simulink model "COSTEP_Exergy"  (R2024b)
settings: Solver=FixedStepAuto  StartTime=0.0  StopTime=25  FixedStep=1/3600  RelTol=1e-3
model workspace (MAT data in the model file):
  AD : Simulink.Parameter (value not decoded)
  AG : Simulink.Parameter (value not decoded)
  AH : Simulink.Parameter (value not decoded)
  AV : Simulink.Parameter (value not decoded)
  AVP : Simulink.Parameter (value not decoded)
  BCHL : Simulink.Parameter (value not decoded)
  BCHV : Simulink.Parameter (value not decoded)
  BD : Simulink.Parameter (value not decoded)
  BDIST : Simulink.Parameter (value not decoded)
  BG : Simulink.Parameter (value not decoded)
  BH : Simulink.Parameter (value not decoded)
  BVP : Simulink.Parameter (value not decoded)
  CD : Simulink.Parameter (value not decoded)
  CDIST : Simulink.Parameter (value not decoded)
  CG : Simulink.Parameter (value not decoded)
  CH : Simulink.Parameter (value not decoded)
  CVP : Simulink.Parameter (value not decoded)
  DDIST : Simulink.Parameter (value not decoded)
  DIST_CONST : Simulink.Parameter (value not decoded)
  ISV : Simulink.Parameter (value not decoded)
  TLAST : Simulink.Parameter (value not decoded)
  TNEXT : Simulink.Parameter (value not decoded)
  XMW : Simulink.Parameter (value not decoded)
  XNS : Simulink.Parameter (value not decoded)
  XNS2 : Simulink.Parameter (value not decoded)
  XNS3 : Simulink.Parameter (value not decoded)
  XNSADD : Simulink.Parameter (value not decoded)
  XNSE : Simulink.Parameter (value not decoded)
symbols that are objects in the model workspace (value not decoded): AD, AG, AH, AV, AVP, BD, BG, BH, BVP, CD, CG, CH, CVP, XMW, XNS, XNS2, XNS3, XNSE
undefined symbols (not defined in the file or in its folder): magnitude, msgbox, SETPT, XMEAS, XMV
libraries: mylib x403, dspindex x31
(part 2 of 13)

== system COSTEP_Exergy/Condenser/Position of Valve 11 % ==
  Bus Selector : BusSelector  OutputSignals=XMV(11)
  Bus Selector1 : BusSelector  OutputSignals=IDV(15)
  Constant : Constant  Value=49
  Control valve : mylib/Control valve  SystemSampleTime=-1  VariantActivationTime=update diagram  AllowFlexibleInterface=on  Latency=0  AutoFrameSizeCalculation=off
  Divide : Product  Inputs=*/
  Initial state variable : mylib/Initial state variable
  Integration : mylib/Integration  SystemSampleTime=-1  VariantActivationTime=update diagram  AllowFlexibleInterface=on  Latency=0  AutoFrameSizeCalculation=off
  Subtract : Sum  Inputs=+-
  VTAU(11) : Constant  Value=5/3600
  "YY(49) " : Outport  PortDimensions=1  VectorParamsAs1DForOutWhenUnconnected=off
  wires:
  Integration/1 -> "YY(49) "/1, Subtract/2  "VPOS(11)"
  Subtract/1 -> Divide/1
  Control valve/1 -> Subtract/1
  VTAU(11)/1 -> Divide/2
  Divide/1 -> Integration/1
  Initial state variable/1 -> Integration/2
  [XMV] -> Bus Selector/1
  Bus Selector/1 -> Control valve/1  "<XMV(11)>"
  Bus Selector1/1 -> Control valve/2  "<IDV(15)>"
  [IDV] -> Bus Selector1/1
  Constant/1 -> Initial state variable/1

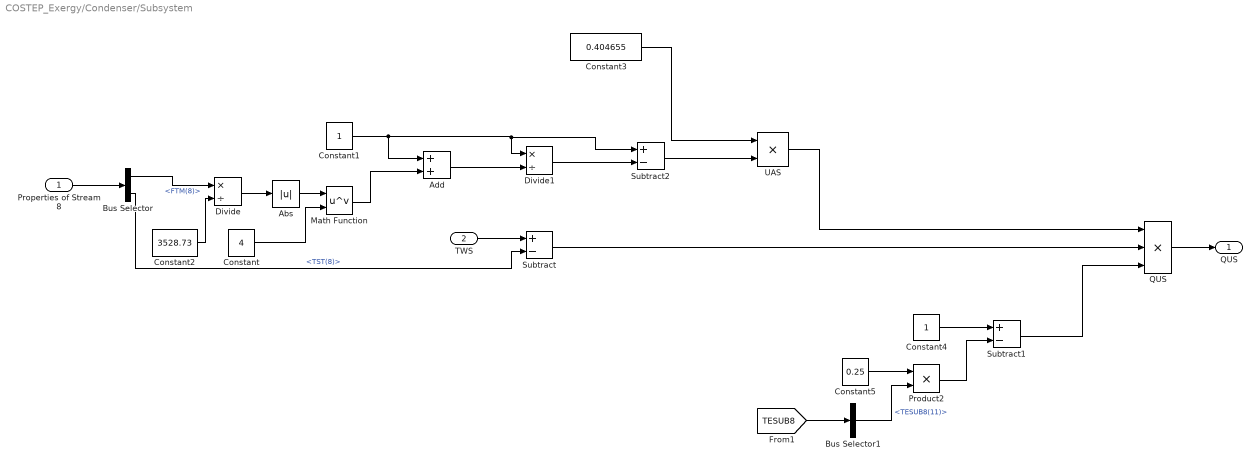
== system COSTEP_Exergy/Condenser/Subsystem ==
  Properties of Stream 8 : Inport
  TWS : Inport  Port=2
  Abs : Abs  SaturateOnIntegerOverflow=off
  Add : Sum
  Bus Selector : BusSelector  OutputSignals=FTM(8),TST(8)
  Bus Selector1 : BusSelector  OutputSignals=signal2.TESUB8(11)
  Constant : Constant  Value=4
  Constant1 : Constant
  Constant2 : Constant  Value=3528.73
  Constant3 : Constant  Value=0.404655
  Constant4 : Constant
  Constant5 : Constant  Value=0.25
  Divide : Product  Inputs=*/
  Divide1 : Product  Inputs=*/
  Math Function : Math  Operator=pow  SignedPower=on
  Product2 : Product
  QUS : Product  Inputs=3
  Subtract : Sum  Inputs=+-
  Subtract1 : Sum  Inputs=+-
  Subtract2 : Sum  Inputs=+-
  UAS : Product
  "QUS " : Outport  VectorParamsAs1DForOutWhenUnconnected=off
  wires:
  Product2/1 -> Subtract1/2
  Constant4/1 -> Subtract1/1
  UAS/1 -> QUS/1
  Properties of Stream 8/1 -> Bus Selector/1
  Add/1 -> Divide1/2
  Constant2/1 -> Divide/2
  Math Function/1 -> Add/2
  Constant1/1 -> Subtract2/1, Divide1/1, Add/1
  Subtract1/1 -> QUS/3
  Constant/1 -> Math Function/2
  Bus Selector/2 -> Subtract/2  "<TST(8)>"
  Bus Selector/1 -> Divide/1  "<FTM(8)>"
  Divide1/1 -> Subtract2/2
  Divide/1 -> Abs/1
  Subtract/1 -> QUS/2
  Constant3/1 -> UAS/1
  Bus Selector1/1 -> Product2/2  "<TESUB8(11)>"
  Subtract2/1 -> UAS/2
  Constant5/1 -> Product2/1
  Abs/1 -> Math Function/1
  [TESUB8] -> Bus Selector1/1
  TWS/1 -> Subtract/1
  QUS/1 -> "QUS "/1

== system COSTEP_Exergy/Condenser/VRNG(11) Max flow of water through valve Gallons per minute ==
  Bus Selector : BusSelector  OutputSignals=signal3.TESUB8(20)
  VRNG(11) : Outport  PortDimensions=1  VectorParamsAs1DForOutWhenUnconnected=off
  wires:
  [TESUB8] -> Bus Selector/1
  Bus Selector/1 -> VRNG(11)/1  "<TESUB8(20)>"

== system COSTEP_Exergy/Control Mode/Braatz ==
  XMEAS : Inport
  " " : Subsystem  mask{Parameter1=XMV(1), Parameter2=XMEAS(2), SETPT1=3664.0, GAIN1=1, SI1=3/3600, HIGH1=5811, Parameter1_copy=SETPT(1), Parameter2_copy=XMEAS(26), SETPT14=6.8820, GAIN14=8.3, TAUI14=3168.0/3600, SI14=360/3600, HIGH14=100}
      mask prompts: Parameter1 "Manipulated Variable"; Parameter2 "Process Variable"; SETPT1 "Setpoint"; GAIN1 "Controller Gain"; SI1 "Sampling Interval"; HIGH1 "High Limit"; Parameter1_copy "Manipulated Variable"; Parameter2_copy "Process Variable"; SETPT14 "Setpoint"; GAIN14 "Controller Gain"; TAUI14 "Integral Time Constant"; SI14 "Sampling Interval"; HIGH14 "High Limit"
      mask DialogControl DescGroupVar Prompt: Control Variables
      mask DialogControl DescTextVar Prompt: Enter the control variables needed
      mask DialogControl ParameterGroupVar Prompt: Control 1
      mask DialogControl Container3 Prompt: Control 14
  " 1" : Subsystem  mask{Parameter1=XMV(2), Parameter2=XMEAS(3), SETPT2=4509.3, GAIN2=1.0, SI2=3/3600, HIGH2=8354, Parameter1_copy=SETPT(2), Parameter2_copy=XMEAS(27), SETPT15=18.776, GAIN15=2.37, TAUI15=5069/3600, SI15=360/3600, HIGH15=100}
      mask prompts: Parameter1 "Manipulated Variable"; Parameter2 "Process Variable"; SETPT2 "Setpoint"; GAIN2 "Controller Gain"; SI2 "Sampling Interval"; HIGH2 "High Limit"; Parameter1_copy "Manipulated Variable"; Parameter2_copy "Process Variable"; SETPT15 "Setpoint"; GAIN15 "Controller Gain"; TAUI15 "Integral Time Constant"; SI15 "Sampling Interval"; HIGH15 "High Limit"
      mask DialogControl DescGroupVar Prompt: Control Variables
      mask DialogControl DescTextVar Prompt: Enter the control variables needed
      mask DialogControl ParameterGroupVar Prompt: Control 2
      mask DialogControl Container3 Prompt: Control 15
  " 10" : Subsystem  mask{Parameter1=XMV(6), Parameter2=XMEAS(10), SETPT6=0.33712, GAIN6=1.22, SI6=3/3600, HIGH6=1, Parameter1_copy=SETPT(6), Parameter2_copy=XMEAS(30), SETPT19=13.823, GAIN19=-83.2/5/3, TAUI19=6336/3600, SI19=360/3600, HIGH19=26}
      mask prompts: Parameter1 "Manipulated Variable"; Parameter2 "Process Variable"; SETPT6 "Setpoint"; GAIN6 "Controller Gain"; SI6 "Sampling Interval"; HIGH6 "High Limit"; Parameter1_copy "Manipulated Variable"; Parameter2_copy "Process Variable"; SETPT19 "Setpoint"; GAIN19 "Controller Gain"; TAUI19 "Integral Time Constant"; SI19 "Sampling Interval"; HIGH19 "High Limit"
      mask DialogControl DescGroupVar Prompt: Control Variables
      mask DialogControl DescTextVar Prompt: Enter the control variables needed
      mask DialogControl ParameterGroupVar Prompt: Control 6
      mask DialogControl Container3 Prompt: Control 19
  " 2" : Subsystem  mask{Parameter1=XMV(3), Parameter2=XMEAS(1), SETPT3=0.25052, GAIN3=1.0, SI3=3/3600, HIGH3=1.017, Parameter1_copy=SETPT(3), Parameter2_copy=XMEAS(23), SETPT13=32.188, GAIN13=18, TAUI13=3168.0/3600, SI13=360/3600, HIGH13=100}
      mask prompts: Parameter1 "Manipulated Variable"; Parameter2 "Process Variable"; SETPT3 "Setpoint"; GAIN3 "Controller Gain"; SI3 "Sampling Interval"; HIGH3 "High Limit"; Parameter1_copy "Manipulated Variable"; Parameter2_copy "Process Variable"; SETPT13 "Setpoint"; GAIN13 "Controller Gain"; TAUI13 "Integral Time Constant"; SI13 "Sampling Interval"; HIGH13 "High Limit"
      mask DialogControl DescGroupVar Prompt: Control Variables
      mask DialogControl DescTextVar Prompt: Enter the control variables needed
      mask DialogControl ParameterGroupVar Prompt: Control 3
      mask DialogControl Container3 Prompt: Control 13
  " 3" : Subsystem  mask{Parameter1=XMV(4), Parameter2=XMEAS(4), SETPT4=9.3477, GAIN4=1.0, SI4=3/3600, HIGH4=15.25, Parameter1_copy=SETPT(4), Parameter2_copy=XMEAS(8), SETPT17=75, GAIN17=11.1/10, TAUI17=3168.0/3600, SI17=3/3600, HIGH17=50}
      mask prompts: Parameter1 "Manipulated Variable"; Parameter2 "Process Variable"; SETPT4 "Setpoint"; GAIN4 "Controller Gain"; SI4 "Sampling Interval"; HIGH4 "High Limit"; Parameter1_copy "Manipulated Variable"; Parameter2_copy "Process Variable"; SETPT17 "Setpoint"; GAIN17 "Controller Gain"; TAUI17 "Integral Time Constant"; SI17 "Sampling Interval"; HIGH17 "High Limit"
      mask DialogControl DescGroupVar Prompt: Control Variables
      mask DialogControl DescTextVar Prompt: Enter the control variables needed
      mask DialogControl ParameterGroupVar Prompt: Control 4
      mask DialogControl Container3 Prompt: Control 17
  " 4" : Subsystem  mask{Parameter1_copy=XMV(5), Parameter2_copy=XMEAS(5), SETPT5=26.902, GAIN5=-0.083, TAUI5=1/3600, SI5=3/3600, HIGH5=53}
      mask prompts: Parameter1_copy "Manipulated Variable"; Parameter2_copy "Process Variable"; SETPT5 "Setpoint"; GAIN5 "Controller Gain"; TAUI5 "Integral Time Constant"; SI5 "Sampling Interval"; HIGH5 "High Limit"
      mask DialogControl DescGroupVar Prompt: Control Variables
      mask DialogControl DescTextVar Prompt: Enter the control variables needed
      mask DialogControl Container3 Prompt: Control 5
  " 5" : Subsystem  mask{Parameter1_copy=XMV(7), Parameter2_copy=XMEAS(12), SETPT7=50, GAIN7=-2.06, SI7=3/3600, HIGH7=70}
      mask prompts: Parameter1_copy "Manipulated Variable"; Parameter2_copy "Process Variable"; SETPT7 "Setpoint"; GAIN7 "Controller Gain"; SI7 "Sampling Interval"; HIGH7 "High Limit"
      mask DialogControl DescGroupVar Prompt: Control Variables
      mask DialogControl DescTextVar Prompt: Enter the control variables needed
      mask DialogControl Container3 Prompt: Control 7
  " 6" : Subsystem  mask{Parameter1_copy=XMV(8), Parameter2_copy=XMEAS(15), SETPT8=50, GAIN8=-1.62, SI8=3/3600, HIGH8=70}
      mask prompts: Parameter1_copy "Manipulated Variable"; Parameter2_copy "Process Variable"; SETPT8 "Setpoint"; GAIN8 "Controller Gain"; SI8 "Sampling Interval"; HIGH8 "High Limit"
      mask DialogControl DescGroupVar Prompt: Control Variables
      mask DialogControl DescTextVar Prompt: Enter the control variables needed
      mask DialogControl Container3 Prompt: Control 8
  " 7" : Subsystem  mask{Parameter1_copy=XMV(11), Parameter2_copy=XMEAS(17), SETPT11=22.949, GAIN11=1.09, TAUI11=2600/3600, SI11=3/3600, HIGH11=46}
      mask prompts: Parameter1_copy "Manipulated Variable"; Parameter2_copy "Process Variable"; SETPT11 "Setpoint"; GAIN11 "Controller Gain"; TAUI11 "Integral Time Constant"; SI11 "Sampling Interval"; HIGH11 "High Limit"
      mask DialogControl DescGroupVar Prompt: Control Variables
      mask DialogControl DescTextVar Prompt: Enter the control variables needed
      mask DialogControl Container3 Prompt: Control 11
  " 8" : Subsystem  mask{Parameter1=XMV(10), Parameter2=XMEAS(21), SETPT10=94.599, GAIN10=-0.156*10, TAUI10=1452/3600, SI10=3/3600, HIGH10=150, Parameter1_copy=SETPT(10), Parameter2_copy=XMEAS(9), SETPT18=120.4, GAIN18=2.83*10, TAUI18=982/3600, SI18=3/3600, HIGH18=150}
      mask prompts: Parameter1 "Manipulated Variable"; Parameter2 "Process Variable"; SETPT10 "Setpoint"; GAIN10 "Controller Gain"; TAUI10 "Integral Time Constant"; SI10 "Sampling Interval"; HIGH10 "High Limit"; Parameter1_copy "Manipulated Variable"; Parameter2_copy "Process Variable"; SETPT18 "Setpoint"; GAIN18 "Controller Gain"; TAUI18 "Integral Time Constant"; SI18 "Sampling Interval"; HIGH18 "High Limit"
      mask DialogControl DescGroupVar Prompt: Control Variables
      mask DialogControl DescTextVar Prompt: Enter the control variables needed
      mask DialogControl ParameterGroupVar Prompt: Control 10
      mask DialogControl Container3 Prompt: Control 18
  " 9" : Subsystem  mask{Parameter1=XMV(9), Parameter2=XMEAS(19), SETPT9=230.31, GAIN9=0.41, SI9=3/3600, HIGH9=460, Parameter1_copy=SETPT(9), Parameter2_copy=XMEAS(18), SETPT16=65.731, GAIN16=1.69/10, TAUI16=236/3600, SI16=3/3600, HIGH16=130, Parameter1_copy_copy=SETPT(16), Parameter2_copy_copy=XMEAS(38), SETPT20=0.83570, GAIN20=-16.3/5, TAUI20=12408/3600, SI20=900/3600, HIGH20=1.6}
      mask prompts: Parameter1 "Manipulated Variable"; Parameter2 "Process Variable"; SETPT9 "Setpoint"; GAIN9 "Controller Gain"; SI9 "Sampling Interval"; HIGH9 "High Limit"; Parameter1_copy "Manipulated Variable"; Parameter2_copy "Process Variable"; SETPT16 "Setpoint"; GAIN16 "Controller Gain"; TAUI16 "Integral Time Constant"; SI16 "Sampling Interval"; HIGH16 "High Limit"; Parameter1_copy_copy "Manipulated Variable"; Parameter2_copy_copy "Process Variable"; SETPT20 "Setpoint"; GAIN20 "Controller Gain"; TAUI20 "Integral Time Constant"; SI20 "Sampling Interval"; HIGH20 "High Limit"
      mask DialogControl DescGroupVar Prompt: Control Variables
      mask DialogControl DescTextVar Prompt: Enter the control variables needed
      mask DialogControl ParameterGroupVar Prompt: Control 9
      mask DialogControl Container3 Prompt: Control 16
      mask DialogControl Container3_copy Prompt: Control 20
  Bus Creator : BusCreator  Inputs=12
  Constant11 : Constant  Value=XMV12_0
  XMV : Outport  VectorParamsAs1DForOutWhenUnconnected=off
  wires:
  " "/1(XMV(1)) -> Bus Creator/1  "XMV(1)"
  " 1"/1(XMV(2)) -> Bus Creator/2  "XMV(2)"
  " 2"/1(XMV(3)) -> Bus Creator/3  "XMV(3)"
  " 3"/1(XMV(4)) -> Bus Creator/4  "XMV(4)"
  " 4"/1(XMV(5)) -> Bus Creator/5  "XMV(5)"
  " 10"/1(XMV(6)) -> Bus Creator/6  "XMV(6)"
  " 5"/1(XMV(7)) -> Bus Creator/7  "XMV(7)"
  " 6"/1(XMV(8)) -> Bus Creator/8  "XMV(8)"
  " 9"/1(XMV(9)) -> Bus Creator/9  "XMV(9)"
  " 8"/1(XMV(10)) -> Bus Creator/10  "XMV(10)"
  " 7"/1(XMV(11)) -> Bus Creator/11  "XMV(11)"
  Constant11/1 -> Bus Creator/12  "XMV(12)"
  Bus Creator/1 -> XMV/1
  XMEAS/1 -> " 5"/1(XMEAS), " 9"/1(XMEAS), " 8"/1(XMEAS), " 7"/1(XMEAS), " 6"/1(XMEAS), " 10"/1(XMEAS), " 4"/1(XMEAS), " 3"/1(XMEAS), " 2"/1(XMEAS), " 1"/1(XMEAS), " "/1(XMEAS)

== system COSTEP_Exergy/Control Mode/Custom Controller ==
  Bus Creator : BusCreator  Inputs=12
  Constant : Constant  Value=XMV1_0
  Constant1 : Constant  Value=XMV2_0
  Constant10 : Constant  Value=XMV11_0
  Constant11 : Constant  Value=XMV12_0
  Constant2 : Constant  Value=XMV3_0
  Constant3 : Constant  Value=XMV4_0
  Constant4 : Constant  Value=XMV5_0
  Constant5 : Constant  Value=XMV6_0
  Constant6 : Constant  Value=XMV7_0
  Constant7 : Constant  Value=XMV8_0
  Constant8 : Constant  Value=XMV9_0
  Constant9 : Constant  Value=XMV10_0
  XMV : Outport  VectorParamsAs1DForOutWhenUnconnected=off
  wires:
  Constant5/1 -> Bus Creator/6  "XMV(6)"
  Constant1/1 -> Bus Creator/2  "XMV(2)"
  Constant4/1 -> Bus Creator/5  "XMV(5)"
  Constant3/1 -> Bus Creator/4  "XMV(4)"
  Constant2/1 -> Bus Creator/3  "XMV(3)"
  Constant11/1 -> Bus Creator/12  "XMV(12)"
  Constant10/1 -> Bus Creator/11  "XMV(11)"
  Constant/1 -> Bus Creator/1  "XMV(1)"
  Constant9/1 -> Bus Creator/10  "XMV(10)"
  Constant8/1 -> Bus Creator/9  "XMV(9)"
  Constant6/1 -> Bus Creator/7  "XMV(7)"
  Bus Creator/1 -> XMV/1
  Constant7/1 -> Bus Creator/8  "XMV(8)"

== system COSTEP_Exergy/Control Mode/Custom Controller1 ==
  Bus Creator : BusCreator  Inputs=12
  Constant : Constant  Value=XMV1_0
  Constant1 : Constant  Value=XMV2_0
  Constant10 : Constant  Value=XMV11_0
  Constant11 : Constant  Value=XMV12_0
  Constant2 : Constant  Value=XMV3_0
  Constant3 : Constant  Value=XMV4_0
  Constant4 : Constant  Value=XMV5_0
  Constant5 : Constant  Value=XMV6_0
  Constant6 : Constant  Value=XMV7_0
  Constant7 : Constant  Value=XMV8_0
  Constant8 : Constant  Value=XMV9_0
  Constant9 : Constant  Value=XMV10_0
  XMV : Outport  VectorParamsAs1DForOutWhenUnconnected=off
  wires:
  Constant5/1 -> Bus Creator/6  "XMV(6)"
  Constant1/1 -> Bus Creator/2  "XMV(2)"
  Constant4/1 -> Bus Creator/5  "XMV(5)"
  Constant3/1 -> Bus Creator/4  "XMV(4)"
  Constant2/1 -> Bus Creator/3  "XMV(3)"
  Constant11/1 -> Bus Creator/12  "XMV(12)"
  Constant10/1 -> Bus Creator/11  "XMV(11)"
  Constant/1 -> Bus Creator/1  "XMV(1)"
  Constant9/1 -> Bus Creator/10  "XMV(10)"
  Constant8/1 -> Bus Creator/9  "XMV(9)"
  Constant6/1 -> Bus Creator/7  "XMV(7)"
  Bus Creator/1 -> XMV/1
  Constant7/1 -> Bus Creator/8  "XMV(8)"

== system COSTEP_Exergy/Control Mode/If Action Subsystem ==
  In1 : Inport
  Action Port : ActionPort  ActionPortLabel=if(u1 == 1)
  Out1 : Outport  VectorParamsAs1DForOutWhenUnconnected=off
  wires:
  In1/1 -> Out1/1

== system COSTEP_Exergy/Control Mode/If Action Subsystem1 ==
  In1 : Inport
  Action Port : ActionPort  ActionPortLabel=elseif(u2 == 1)
  Out1 : Outport  VectorParamsAs1DForOutWhenUnconnected=off
  wires:
  In1/1 -> Out1/1

== system COSTEP_Exergy/Control Mode/If Action Subsystem2 ==
  In1 : Inport
  Action Port : ActionPort  ActionPortLabel=elseif( u3 == 1)
  Out1 : Outport  VectorParamsAs1DForOutWhenUnconnected=off
  wires:
  In1/1 -> Out1/1

== system COSTEP_Exergy/Control Mode/If Action Subsystem3 ==
  XMV : Inport
  Action Port : ActionPort  ActionPortLabel=elseif( u4 == 1)
  Out1 : Outport  VectorParamsAs1DForOutWhenUnconnected=off
  wires:
  XMV/1 -> Out1/1

== system COSTEP_Exergy/Control Mode/Open loop ==
  Bus Creator : BusCreator  Inputs=12
  Constant : Constant  Value=XMV1_0
  Constant1 : Constant  Value=XMV2_0
  Constant10 : Constant  Value=XMV11_0
  Constant11 : Constant  Value=XMV12_0
  Constant2 : Constant  Value=XMV3_0
  Constant3 : Constant  Value=XMV4_0
  Constant4 : Constant  Value=XMV5_0
  Constant5 : Constant  Value=XMV6_0
  Constant6 : Constant  Value=XMV7_0
  Constant7 : Constant  Value=XMV8_0
  Constant8 : Constant  Value=XMV9_0
  Constant9 : Constant  Value=XMV10_0
  XMV : Outport  VectorParamsAs1DForOutWhenUnconnected=off
  wires:
  Constant5/1 -> Bus Creator/6  "XMV(6)"
  Constant1/1 -> Bus Creator/2  "XMV(2)"
  Constant4/1 -> Bus Creator/5  "XMV(5)"
  Constant3/1 -> Bus Creator/4  "XMV(4)"
  Constant2/1 -> Bus Creator/3  "XMV(3)"
  Constant11/1 -> Bus Creator/12  "XMV(12)"
  Constant10/1 -> Bus Creator/11  "XMV(11)"
  Constant/1 -> Bus Creator/1  "XMV(1)"
  Constant9/1 -> Bus Creator/10  "XMV(10)"
  Constant8/1 -> Bus Creator/9  "XMV(9)"
  Constant6/1 -> Bus Creator/7  "XMV(7)"
  Bus Creator/1 -> XMV/1
  Constant7/1 -> Bus Creator/8  "XMV(8)"

== system COSTEP_Exergy/Control Mode/Subsystem ==
  OPL : Inport
  B : Inport  Port=2
  R : Inport  Port=3
  C : Inport  Port=4
  Assertion : Assertion  AssertionFailFcn=|  StopWhenAssertionFail=off
      | set_param(bdroot,'SimulationCommand','stop'),
      | disp(sprintf('\nSimulation stoped.')), msgbox({'Simulation will not run';'More than one loop selected'}, 'Shutdown','error')
  Constant3 : Constant  Value=2
  Relational Operator : RelationalOperator  Operator=<  OutDataTypeStr=boolean  RndMeth=Simplest  InputSameDT=off
  Sum of Elements : Sum  Inputs=++++
  wires:
  Sum of Elements/1 -> Relational Operator/1
  R/1 -> Sum of Elements/3
  OPL/1 -> Sum of Elements/1
  Relational Operator/1 -> Assertion/1
  Constant3/1 -> Relational Operator/2
  B/1 -> Sum of Elements/2
  C/1 -> Sum of Elements/4

== system COSTEP_Exergy/D Feed Stream/HST(1) Molar Enthalpy of Stream 1 MBtu//lb-mol ==
  TST(1) : Inport
  XST(I,1) : Inport  Port=2
  "Enthalpy of Stream " : mylib/Enthalpy of Stream   SystemSampleTime=-1  VariantActivationTime=update diagram  AllowFlexibleInterface=on  Latency=0  AutoFrameSizeCalculation=off
  ITY : Constant
  HST(1) : Outport  VectorParamsAs1DForOutWhenUnconnected=off
  wires:
  ITY/1 -> "Enthalpy of Stream "/1
  TST(1)/1 -> "Enthalpy of Stream "/2
  XST(I,1)/1 -> "Enthalpy of Stream "/3
  "Enthalpy of Stream "/1 -> HST(1)/1

== system COSTEP_Exergy/D Feed Stream/TST(1) Temperature of Stream 1 °C ==
  Add : Sum
  Bus Selector : BusSelector  OutputSignals=signal1.TESUB8(3)
  Bus Selector1 : BusSelector  OutputSignals=IDV(3)
  Gain : Gain  Gain=5
  TST(1) : Outport  PortDimensions=1  VectorParamsAs1DForOutWhenUnconnected=off
  wires:
  Bus Selector1/1 -> Gain/1  "<IDV(3)>"
  [IDV] -> Bus Selector1/1
  [TESUB8] -> Bus Selector/1
  Add/1 -> TST(1)/1  "TST(1)"
  Gain/1 -> Add/2
  Bus Selector/1 -> Add/1  "<TESUB8(3)>"

== system COSTEP_Exergy/D Feed Stream/VRNG(1) Max flow of Stream 1 through valve lb-mol//h ==
  Bus Selector : BusSelector  OutputSignals=signal3.TESUB8(16)
  VRNG(1) : Outport  PortDimensions=1  VectorParamsAs1DForOutWhenUnconnected=off
  wires:
  [TESUB8] -> Bus Selector/1
  Bus Selector/1 -> VRNG(1)/1  "<TESUB8(16)>"

== system COSTEP_Exergy/Disturbances/IDV bus signal ==
  IDV : Inport
  Bus Creator : BusCreator  Inputs=28
  Demux : Demux  Outputs=28
  Out1 : Outport
  wires:
  Demux/5 -> Bus Creator/5  "IDV(5)"
  Demux/4 -> Bus Creator/4  "IDV(4)"
  Demux/2 -> Bus Creator/2  "IDV(2)"
  Demux/12 -> Bus Creator/12  "IDV(12)"
  Demux/8 -> Bus Creator/8  "IDV(8)"
  Demux/9 -> Bus Creator/9  "IDV(9)"
  Demux/14 -> Bus Creator/14  "IDV(14)"
  Demux/20 -> Bus Creator/20  "IDV(20)"
  Demux/16 -> Bus Creator/16  "IDV(16)"
  Demux/6 -> Bus Creator/6  "IDV(6)"
  Demux/13 -> Bus Creator/13  "IDV(13)"
  Demux/1 -> Bus Creator/1  "IDV(1)"
  Demux/19 -> Bus Creator/19  "IDV(19)"
  Demux/3 -> Bus Creator/3  "IDV(3)"
  Demux/10 -> Bus Creator/10  "IDV(10)"
  Demux/18 -> Bus Creator/18  "IDV(18)"
  Demux/17 -> Bus Creator/17  "IDV(17)"
  Demux/15 -> Bus Creator/15  "IDV(15)"
  Demux/11 -> Bus Creator/11  "IDV(11)"
  Demux/7 -> Bus Creator/7  "IDV(7)"
  Bus Creator/1 -> Out1/1
  Demux/21 -> Bus Creator/21  "IDV(21)"
  Demux/22 -> Bus Creator/22  "IDV(22)"
  Demux/23 -> Bus Creator/23  "IDV(23)"
  Demux/24 -> Bus Creator/24  "IDV(24)"
  Demux/25 -> Bus Creator/25  "IDV(25)"
  Demux/26 -> Bus Creator/26  "IDV(26)"
  Demux/27 -> Bus Creator/27  "IDV(27)"
  Demux/28 -> Bus Creator/28  "IDV(28)"
  IDV/1 -> Demux/1

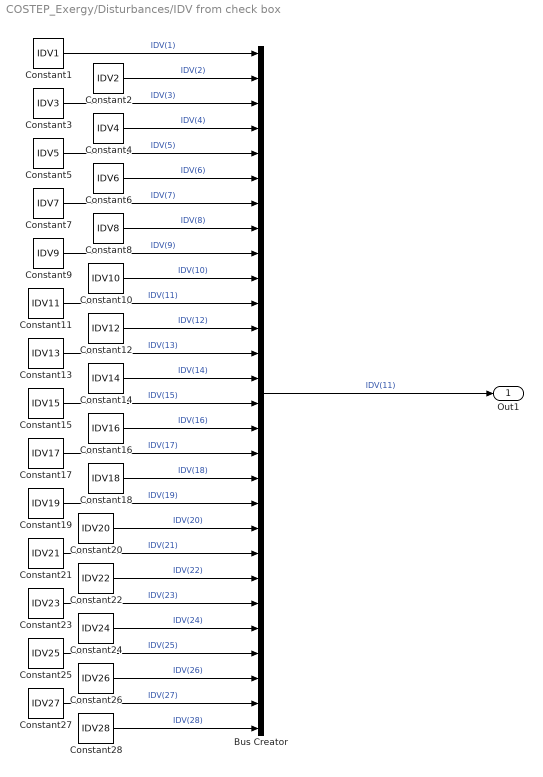
== system COSTEP_Exergy/Disturbances/IDV from check box ==
  Bus Creator : BusCreator  Inputs=28
  Constant1 : Constant  Value=IDV1
  Constant10 : Constant  Value=IDV10
  Constant11 : Constant  Value=IDV11
  Constant12 : Constant  Value=IDV12
  Constant13 : Constant  Value=IDV13
  Constant14 : Constant  Value=IDV14
  Constant15 : Constant  Value=IDV15
  Constant16 : Constant  Value=IDV16
  Constant17 : Constant  Value=IDV17
  Constant18 : Constant  Value=IDV18
  Constant19 : Constant  Value=IDV19
  Constant2 : Constant  Value=IDV2
  Constant20 : Constant  Value=IDV20
  Constant21 : Constant  Value=IDV21
  Constant22 : Constant  Value=IDV22
  Constant23 : Constant  Value=IDV23
  Constant24 : Constant  Value=IDV24
  Constant25 : Constant  Value=IDV25
  Constant26 : Constant  Value=IDV26
  Constant27 : Constant  Value=IDV27
  Constant28 : Constant  Value=IDV28
  Constant3 : Constant  Value=IDV3
  Constant4 : Constant  Value=IDV4
  Constant5 : Constant  Value=IDV5
  Constant6 : Constant  Value=IDV6
  Constant7 : Constant  Value=IDV7
  Constant8 : Constant  Value=IDV8
  Constant9 : Constant  Value=IDV9
  Out1 : Outport
  wires:
  Constant5/1 -> Bus Creator/5  "IDV(5)"
  Constant4/1 -> Bus Creator/4  "IDV(4)"
  Constant2/1 -> Bus Creator/2  "IDV(2)"
  Constant12/1 -> Bus Creator/12  "IDV(12)"
  Constant8/1 -> Bus Creator/8  "IDV(8)"
  Constant9/1 -> Bus Creator/9  "IDV(9)"
  Constant14/1 -> Bus Creator/14  "IDV(14)"
  Constant20/1 -> Bus Creator/20  "IDV(20)"
  Constant16/1 -> Bus Creator/16  "IDV(16)"
  Constant6/1 -> Bus Creator/6  "IDV(6)"
  Constant13/1 -> Bus Creator/13  "IDV(13)"
  Constant1/1 -> Bus Creator/1  "IDV(1)"
  Constant19/1 -> Bus Creator/19  "IDV(19)"
  Constant3/1 -> Bus Creator/3  "IDV(3)"
  Constant10/1 -> Bus Creator/10  "IDV(10)"
  Constant18/1 -> Bus Creator/18  "IDV(18)"
  Constant17/1 -> Bus Creator/17  "IDV(17)"
  Constant15/1 -> Bus Creator/15  "IDV(15)"
  Constant11/1 -> Bus Creator/11  "IDV(11)"
  Constant7/1 -> Bus Creator/7  "IDV(7)"
  Constant21/1 -> Bus Creator/21  "IDV(21)"
  Constant22/1 -> Bus Creator/22  "IDV(22)"
  Constant23/1 -> Bus Creator/23  "IDV(23)"
  Constant24/1 -> Bus Creator/24  "IDV(24)"
  Constant25/1 -> Bus Creator/25  "IDV(25)"
  Constant26/1 -> Bus Creator/26  "IDV(26)"
  Constant27/1 -> Bus Creator/27  "IDV(27)"
  Constant28/1 -> Bus Creator/28  "IDV(28)"
  Bus Creator/1 -> Out1/1  "IDV(11)"

== system COSTEP_Exergy/E Feed Stream/HST(2) Molar Enthalpy of Stream 2 MBtu//lb-mol ==
  TST(2) : Inport
  XST(I,2) : Inport  Port=2
  "Enthalpy of Stream " : mylib/Enthalpy of Stream   SystemSampleTime=-1  VariantActivationTime=update diagram  AllowFlexibleInterface=on  Latency=0  AutoFrameSizeCalculation=off
  ITY : Constant
  HST(2) : Outport  VectorParamsAs1DForOutWhenUnconnected=off
  wires:
  ITY/1 -> "Enthalpy of Stream "/1
  TST(2)/1 -> "Enthalpy of Stream "/2
  XST(I,2)/1 -> "Enthalpy of Stream "/3
  "Enthalpy of Stream "/1 -> HST(2)/1

== system COSTEP_Exergy/E Feed Stream/TST(2) Temperature of Stream 2 °C ==
  Bus Selector : BusSelector  OutputSignals=signal3.TESUB8(14)
  TST(2) : Outport  PortDimensions=1  VectorParamsAs1DForOutWhenUnconnected=off
  wires:
  [TESUB8] -> Bus Selector/1
  Bus Selector/1 -> TST(2)/1  "<TESUB8(14)>"

== system COSTEP_Exergy/E Feed Stream/VRNG(2) Max flow of Stream 2 through valve lb-mol//h ==
  Bus Selector : BusSelector  OutputSignals=signal3.TESUB8(17)
  VRNG(2) : Outport  PortDimensions=1  VectorParamsAs1DForOutWhenUnconnected=off
  wires:
  [TESUB8] -> Bus Selector/1
  Bus Selector/1 -> VRNG(2)/1  "<TESUB8(17)>"

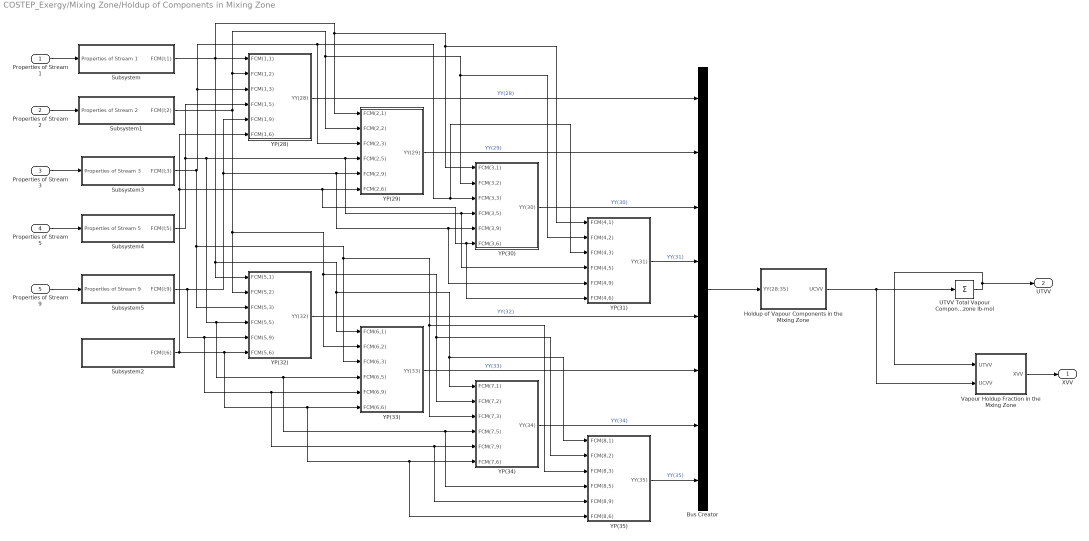
== system COSTEP_Exergy/Mixing Zone/Holdup of Components in Mixing Zone ==
  Properties of Stream 1 : Inport
  Properties of Stream 2 : Inport  Port=2
  Properties of Stream 3 : Inport  Port=3
  Properties of Stream 5 : Inport  Port=4
  Properties of Stream 9 : Inport  Port=5
  Bus Creator : BusCreator  Inputs=8
  Holdup of Vapour Components in the Mixing Zone : Subsystem
  Subsystem : Subsystem
  Subsystem1 : Subsystem
  Subsystem2 : Subsystem
  Subsystem3 : Subsystem
  Subsystem4 : Subsystem
  Subsystem5 : Subsystem
  UTVV Total Vapour Component holdup in Mixing zone lb-mol : Sum  Inputs=+
  Vapour Holdup Fraction in the Mxing Zone : Subsystem
  YP(28) : Subsystem
  YP(29) : Subsystem
  YP(30) : Subsystem
  YP(31) : Subsystem
  YP(32) : Subsystem
  YP(33) : Subsystem
  YP(34) : Subsystem
  YP(35) : Subsystem
  XVV : Outport  PortDimensions=8  VectorParamsAs1DForOutWhenUnconnected=off
  UTVV : Outport  Port=2  PortDimensions=1  VectorParamsAs1DForOutWhenUnconnected=off
  wires:
  YP(28)/1(YY(28)) -> Bus Creator/1  "YY(28)"
  YP(29)/1(YY(29)) -> Bus Creator/2  "YY(29)"
  YP(30)/1(YY(30)) -> Bus Creator/3  "YY(30)"
  YP(31)/1(YY(31)) -> Bus Creator/4  "YY(31)"
  YP(32)/1(YY(32)) -> Bus Creator/5  "YY(32)"
  YP(33)/1(YY(33)) -> Bus Creator/6  "YY(33)"
  YP(34)/1(YY(34)) -> Bus Creator/7  "YY(34)"
  YP(35)/1(YY(35)) -> Bus Creator/8  "YY(35)"
  Bus Creator/1 -> Holdup of Vapour Components in the Mixing Zone/1(YY(28:35))
  Holdup of Vapour Components in the Mixing Zone/1(UCVV) -> Vapour Holdup Fraction in the Mxing Zone/2(UCVV), UTVV Total Vapour Component holdup in Mixing zone lb-mol/1
  UTVV Total Vapour Component holdup in Mixing zone lb-mol/1 -> UTVV/1, Vapour Holdup Fraction in the Mxing Zone/1(UTVV)
  Vapour Holdup Fraction in the Mxing Zone/1(XVV) -> XVV/1
  Properties of Stream 1/1 -> Subsystem/1(Properties of Stream 1)
  Properties of Stream 2/1 -> Subsystem1/1(Properties of Stream 2)
  Properties of Stream 3/1 -> Subsystem3/1(Properties of Stream 3)
  Properties of Stream 5/1 -> Subsystem4/1(Properties of Stream 5)
  Properties of Stream 9/1 -> Subsystem5/1(Properties of Stream 9)
  Subsystem/1(FCM(I;1)) -> YP(35)/1(FCM(8,1)), YP(34)/1(FCM(7,1)), YP(33)/1(FCM(6,1)), YP(32)/1(FCM(5,1)), YP(31)/1(FCM(4,1)), YP(30)/1(FCM(3,1)), YP(29)/1(FCM(2,1)), YP(28)/1(FCM(1,1))
  Subsystem1/1(FCM(I;2)) -> YP(35)/2(FCM(8,2)), YP(34)/2(FCM(7,2)), YP(33)/2(FCM(6,2)), YP(32)/2(FCM(5,2)), YP(31)/2(FCM(4,2)), YP(30)/2(FCM(3,2)), YP(29)/2(FCM(2,2)), YP(28)/2(FCM(1,2))
  Subsystem3/1(FCM(I;3)) -> YP(35)/3(FCM(8,3)), YP(34)/3(FCM(7,3)), YP(33)/3(FCM(6,3)), YP(32)/3(FCM(5,3)), YP(29)/3(FCM(2,3)), YP(31)/3(FCM(4,3)), YP(30)/3(FCM(3,3)), YP(28)/3(FCM(1,3))
  Subsystem4/1(FCM(I;5)) -> YP(35)/4(FCM(8,5)), YP(34)/4(FCM(7,5)), YP(33)/4(FCM(6,5)), YP(32)/4(FCM(5,5)), YP(31)/4(FCM(4,5)), YP(30)/4(FCM(3,5)), YP(29)/4(FCM(2,5)), YP(28)/4(FCM(1,5))
  Subsystem5/1(FCM(I;9)) -> YP(35)/5(FCM(8,9)), YP(34)/5(FCM(7,9)), YP(33)/5(FCM(6,9)), YP(32)/5(FCM(5,9)), YP(31)/5(FCM(4,9)), YP(30)/5(FCM(3,9)), YP(29)/5(FCM(2,9)), YP(28)/5(FCM(1,9))
  Subsystem2/1(FCM(I;6)) -> YP(35)/6(FCM(8,6)), YP(34)/6(FCM(7,6)), YP(33)/6(FCM(6,6)), YP(32)/6(FCM(5,6)), YP(31)/6(FCM(4,6)), YP(30)/6(FCM(3,6)), YP(29)/6(FCM(2,6)), YP(28)/6(FCM(1,6))

== system COSTEP_Exergy/Mixing Zone/Internal energy of mixing zone ==
  Properties of Stream 1 : Inport
  Properties of Stream 2 : Inport  Port=2
  Properties of Stream 3 : Inport  Port=3
  Properties of Stream 5 : Inport  Port=4
  Properties of Stream 9 : Inport  Port=5
  Add : Sum  Inputs=+++++-
  Bus Selector : BusSelector  OutputSignals=HST(1),FTM(1)
  Bus Selector1 : BusSelector  OutputSignals=HST(2),FTM(2)
  Bus Selector2 : BusSelector  OutputSignals=HST(3),FTM(3)
  Bus Selector3 : BusSelector  OutputSignals=HST(5),FTM(5)
  Bus Selector4 : BusSelector  OutputSignals=HST(9),FTM(9)
  Bus Selector5 : BusSelector  OutputSignals=signal1.HST(6) = HST(7),signal1.FTM(6) = FTM(7)
  Constant : Constant  Value=36
  Initial state variable : mylib/Initial state variable
  Integration : mylib/Integration  SystemSampleTime=-1  VariantActivationTime=update diagram  AllowFlexibleInterface=on  Latency=0  AutoFrameSizeCalculation=off
  Product{,1..5} (6 alike) : Product
  "YY(36) " : Outport  VectorParamsAs1DForOutWhenUnconnected=off
  wires:
  Bus Selector/1 -> Product/1  "<HST(1)>"
  Bus Selector/2 -> Product/2  "<FTM(1)>"
  Bus Selector1/2 -> Product1/2  "<FTM(2)>"
  Bus Selector1/1 -> Product1/1  "<HST(2)>"
  Product/1 -> Add/1
  Product1/1 -> Add/2
  Integration/1 -> "YY(36) "/1
  Initial state variable/1 -> Integration/2
  Add/1 -> Integration/1
  Bus Selector3/1 -> Product3/1  "<HST(5)>"
  Bus Selector2/2 -> Product2/2  "<FTM(3)>"
  Product2/1 -> Add/3
  Bus Selector3/2 -> Product3/2  "<FTM(5)>"
  Product3/1 -> Add/4
  Bus Selector2/1 -> Product2/1  "<HST(3)>"
  Bus Selector4/2 -> Product4/2  "<FTM(9)>"
  Bus Selector5/1 -> Product5/1  "<HST(6) = HST(7)>"
  Bus Selector4/1 -> Product4/1  "<HST(9)>"
  Product5/1 -> Add/6
  Product4/1 -> Add/5
  Bus Selector5/2 -> Product5/2  "<FTM(6) = FTM(7)>"
  Properties of Stream 1/1 -> Bus Selector/1
  Properties of Stream 2/1 -> Bus Selector1/1
  Properties of Stream 3/1 -> Bus Selector2/1
  Properties of Stream 5/1 -> Bus Selector3/1
  Properties of Stream 9/1 -> Bus Selector4/1
  [PropertiesStream6] -> Bus Selector5/1
  Constant/1 -> Initial state variable/1

== system COSTEP_Exergy/Mixing Zone/PTV Total pressure of Mixing zone mmHg ==
  UTVV : Inport
  TCV : Inport  Port=2
  PTV Total pressure of Mixing zone mmHg : Product  Inputs=***/
  RG Universal Gas Constant ft³·mmHg/K·lb-mol : Constant  Value=998.9
  TKV Temperature in Mixing zone K : Sum
  To Convert °C to K : Constant  Value=273.15
  VTV Total Volume of Mixing zone ft³ : Constant  Value=5000
  PTV : Outport  VectorParamsAs1DForOutWhenUnconnected=off
  wires:
  RG Universal Gas Constant ft³·mmHg/K·lb-mol/1 -> PTV Total pressure of Mixing zone mmHg/2
  VTV Total Volume of Mixing zone ft³/1 -> PTV Total pressure of Mixing zone mmHg/4
  TKV Temperature in Mixing zone K/1 -> PTV Total pressure of Mixing zone mmHg/3
  TCV/1 -> TKV Temperature in Mixing zone K/1
  PTV Total pressure of Mixing zone mmHg/1 -> PTV/1
  To Convert °C to K/1 -> TKV Temperature in Mixing zone K/2
  UTVV/1 -> PTV Total pressure of Mixing zone mmHg/1

== system COSTEP_Exergy/Mixing Zone/Stream 6 ==
  XST(I,6) : Inport
  TST(6) : Inport  Port=2  PortDimensions=1
  Bus Creator : BusCreator  Inputs=6
  FCM(I,6) Component molar flow of Stream 6 lb-mol/h : Product
  FTM(6) : Product  Inputs=*/
  HST(6) Molar Enthalpy of Stream 6 MBtu/lb-mol : Subsystem
  ITY : Constant
  Subsystem : Subsystem
  XMWS(6) Molecular weight of Stream 6 lb/lb-mol : Subsystem
  Properties of Stream 6 : Outport  VectorParamsAs1DForOutWhenUnconnected=off
  wires:
  XMWS(6) Molecular weight of Stream 6 lb/lb-mol/1(XMWS(6)) -> FTM(6)/2
  ITY/1 -> Bus Creator/6, HST(6) Molar Enthalpy of Stream 6 MBtu/lb-mol/1(ITY)  "Phase"
  XST(I,6)/1 -> Bus Creator/1, HST(6) Molar Enthalpy of Stream 6 MBtu/lb-mol/3(XST(I,6)), FCM(I,6) Component molar flow of Stream 6 lb-mol/h/1, XMWS(6) Molecular weight of Stream 6 lb/lb-mol/1(XST(I,6))  "XST(I;6) = XST(I;7)"
  TST(6)/1 -> Bus Creator/2, HST(6) Molar Enthalpy of Stream 6 MBtu/lb-mol/2(T)  "TST(6) = TST(7)"
  HST(6) Molar Enthalpy of Stream 6 MBtu/lb-mol/1("H ") -> Bus Creator/3  "HST(6) = HST(7)"
  FTM(6)/1 -> FCM(I,6) Component molar flow of Stream 6 lb-mol/h/2, Bus Creator/4  "FTM(6) = FTM(7)"
  FCM(I,6) Component molar flow of Stream 6 lb-mol/h/1 -> Bus Creator/5  "FCM(I;6) = FCM(I;7)"
  Bus Creator/1 -> Properties of Stream 6/1
  Subsystem/1("FLMS ") -> FTM(6)/1

== system COSTEP_Exergy/Mixing Zone/TCV Initial Temperature in Mixing zone °C  ==
  UTVV : Inport
  ETV : Inport  Port=2  PortDimensions=1
  XVV : Inport  Port=3
  "AG(I) Coefficient A to determine Enthalpy MBtu/lb·°F " : Constant  Value=AG
  "AH(I) Coefficient A to determine Enthalpy MBtu/lb·°F " : Constant  Value=AH
  AV(I) Coefficient AV to determine Enthalpy MBtu/lb : Constant  Value=AV
  BG(I) Coefficient B to determine Enthalpy MBtu/lb·°F² : Constant  Value=BG
  BH(I) Coefficient B to determine Enthalpy MBtu/lb·°F² : Constant  Value=BH
  CG(I) Coefficient C to determine Enthalpy MBtu/lb·°F³ : Constant  Value=CG
  CH(I) Coefficient C to determine Enthalpy MBtu/lb·°F³ : Constant  Value=CH
  Delay : Delay  DelayLength=1  InitialCondition=0
  ITY : Constant  Value=2
  MATLAB Function : MATLAB Function  TreatAsAtomicUnit=on
  "XMW(I) Molecular weight of components lb/lb-mol " : Constant  Value=XMW
  TCV : Outport  PortDimensions=1  VectorParamsAs1DForOutWhenUnconnected=off
  wires:
  MATLAB Function/1(TCV) -> TCV/1, Delay/1
  Delay/1 -> MATLAB Function/13("TCV ")
  "AG(I) Coefficient A to determine Enthalpy MBtu/lb·°F "/1 -> MATLAB Function/4(AG)
  AV(I) Coefficient AV to determine Enthalpy MBtu/lb/1 -> MATLAB Function/7(AV)
  ETV/1 -> MATLAB Function/10(ETV)
  CH(I) Coefficient C to determine Enthalpy MBtu/lb·°F³/1 -> MATLAB Function/3(CH)
  UTVV/1 -> MATLAB Function/11(UTVV)
  ITY/1 -> MATLAB Function/12(ITY)
  "XMW(I) Molecular weight of components lb/lb-mol "/1 -> MATLAB Function/8(XMW)
  XVV/1 -> MATLAB Function/9(XVV)
  "AH(I) Coefficient A to determine Enthalpy MBtu/lb·°F "/1 -> MATLAB Function/1(AH)
  CG(I) Coefficient C to determine Enthalpy MBtu/lb·°F³/1 -> MATLAB Function/6(CG)
  BH(I) Coefficient B to determine Enthalpy MBtu/lb·°F²/1 -> MATLAB Function/2(BH)
  BG(I) Coefficient B to determine Enthalpy MBtu/lb·°F²/1 -> MATLAB Function/5(BG)

== system COSTEP_Exergy/Process Measurements/Compressor Work ==
  Add : Sum
  Bus Selector1 : BusSelector  OutputSignals=XMNS(20)
  XMEAS(20) : Gain  Gain=0.29307E3
  "XMEAS(20) " : Outport  VectorParamsAs1DForOutWhenUnconnected=off
  wires:
  [CPDH] -> XMEAS(20)/1
  XMEAS(20)/1 -> Add/1
  Add/1 -> "XMEAS(20) "/1  "XMEAS(20)"
  [XMNS] -> Bus Selector1/1
  Bus Selector1/1 -> Add/2  "<XMNS(20)>"

== system COSTEP_Exergy/Process Measurements/Condenser Cooling Outlet Water Temperature ==
  Add : Sum
  Bus Selector1 : BusSelector  OutputSignals=XMNS(22)
  XMEAS(22) : Outport  PortDimensions=1  VectorParamsAs1DForOutWhenUnconnected=off
  wires:
  [TWS] -> Add/1
  Add/1 -> XMEAS(22)/1  "XMEAS(22)"
  [XMNS] -> Bus Selector1/1
  Bus Selector1/1 -> Add/2  "<XMNS(22)>"

== system COSTEP_Exergy/Process Measurements/Feed Streams ==
  " A Feed" : Subsystem
  A and C Feed : Subsystem
  Bus Creator2 : BusCreator  Inputs=5
  D Feed : Subsystem
  E Feed : Subsystem
  Recycle Flow : Subsystem
  XMEASF : Outport  VectorParamsAs1DForOutWhenUnconnected=off
  wires:
  " A Feed"/1("XMEAS(1) ") -> Bus Creator2/1
  E Feed/1("XMEAS(3) ") -> Bus Creator2/3
  A and C Feed/1("XMEAS(4) ") -> Bus Creator2/4
  Bus Creator2/1 -> XMEASF/1
  D Feed/1("XMEAS(2) ") -> Bus Creator2/2
  Recycle Flow/1("XMEAS(5) ") -> Bus Creator2/5

== system COSTEP_Exergy/Process Measurements/Product analysis ==
  Bus Creator : BusCreator  Inputs=5
  Bus Selector : BusSelector  OutputSignals=XST(I;13)
  Scope : Scope
  Subsystem : Subsystem
  XMEAS : Outport  VectorParamsAs1DForOutWhenUnconnected=off
  wires:
  [PropertiesStream13] -> Bus Selector/1
  Bus Creator/1 -> Scope/1, XMEAS/1
  Bus Selector/1 -> Subsystem/1(<XST(I;13)>)  "<XST(I;13)>"
  Subsystem/1(XMEAS(37)) -> Bus Creator/1  "XMEAS(37)"
  Subsystem/2(XMEAS(38)) -> Bus Creator/2  "XMEAS(38)"
  Subsystem/3(XMEAS(39)) -> Bus Creator/3  "XMEAS(39)"
  Subsystem/4(XMEAS(40)) -> Bus Creator/4  "XMEAS(40)"
  Subsystem/5(XMEAS(41)) -> Bus Creator/5  "XMEAS(41)"

== system COSTEP_Exergy/Process Measurements/Purge gas analysis ==
  Bus Creator : BusCreator  Inputs=8
  Bus Selector : BusSelector  OutputSignals=signal1.XST(I;10)
  Subsystem : Subsystem
  XMEASP : Outport  VectorParamsAs1DForOutWhenUnconnected=off
  wires:
  [PropertiesStream10] -> Bus Selector/1
  Bus Creator/1 -> XMEASP/1
  Bus Selector/1 -> Subsystem/1(<XST(I;10)>)  "<XST(I;10)>"
  Subsystem/1(XMEAS(29)) -> Bus Creator/1  "XMEAS(29)"
  Subsystem/2(XMEAS(30)) -> Bus Creator/2  "XMEAS(30)"
  Subsystem/3(XMEAS(31)) -> Bus Creator/3  "XMEAS(31)"
  Subsystem/4(XMEAS(32)) -> Bus Creator/4  "XMEAS(32)"
  Subsystem/5(XMEAS(33)) -> Bus Creator/5  "XMEAS(33)"
  Subsystem/6(XMEAS(34)) -> Bus Creator/6  "XMEAS(34)"
  Subsystem/7(XMEAS(35)) -> Bus Creator/7  "XMEAS(35)"
  Subsystem/8(XMEAS(36)) -> Bus Creator/8  "XMEAS(36)"

== system COSTEP_Exergy/Process Measurements/Reactor Cooling Outlet Water Temperature ==
  Add : Sum
  Bus Selector1 : BusSelector  OutputSignals=XMNS(21)
  XMEAS(21) : Outport  PortDimensions=1  VectorParamsAs1DForOutWhenUnconnected=off
  wires:
  [TWR] -> Add/1
  Add/1 -> XMEAS(21)/1  "XMEAS(21)"
  [XMNS] -> Bus Selector1/1
  Bus Selector1/1 -> Add/2  "<XMNS(21)>"

== system COSTEP_Exergy/Process Measurements/Reactor feed analysis ==
  Bus Creator : BusCreator  Inputs=6
  Bus Selector : BusSelector  OutputSignals=signal1.XST(I;6) = XST(I;7)
  Subsystem : Subsystem
  XMEASR : Outport  VectorParamsAs1DForOutWhenUnconnected=off
  wires:
  [PropertiesStream6] -> Bus Selector/1
  Bus Creator/1 -> XMEASR/1
  Bus Selector/1 -> Subsystem/1(<XST(I;6) = XST(I;7)>)  "<XST(I;6) = XST(I;7)>"
  Subsystem/1(XMEAS(23)) -> Bus Creator/1  "XMEAS(23)"
  Subsystem/2(XMEAS(24)) -> Bus Creator/2  "XMEAS(24)"
  Subsystem/3(XMEAS(25)) -> Bus Creator/3  "XMEAS(25)"
  Subsystem/4(XMEAS(26)) -> Bus Creator/4  "XMEAS(26)"
  Subsystem/5(XMEAS(27)) -> Bus Creator/5  "XMEAS(27)"
  Subsystem/6(XMEAS(28)) -> Bus Creator/6  "XMEAS(28)"

== system COSTEP_Exergy/Process Measurements/Subsystem3 ==
  Bus Creator : BusCreator  Inputs=4
  "Reactor Feed " : Subsystem
  Reactor Level : Subsystem
  Reactor Pressure : Subsystem
  Reactor Temperature : Subsystem
  Reactor : Outport  VectorParamsAs1DForOutWhenUnconnected=off
  wires:
  Reactor Pressure/1("XMEAS(7) ") -> Bus Creator/2
  Reactor Level/1("XMEAS(8) ") -> Bus Creator/3
  Bus Creator/1 -> Reactor/1
  "Reactor Feed "/1("XMEAS(6) ") -> Bus Creator/1
  Reactor Temperature/1("XMEAS(9) ") -> Bus Creator/4

== system COSTEP_Exergy/Process Measurements/Subsystem4 ==
  Bus Creator3 : BusCreator  Inputs=5
  Purge Rate : Subsystem
  Separator Level : Subsystem
  Separator Pressure : Subsystem
  Separator Temperature : Subsystem
  Separator Underflow : Subsystem
  Separator : Outport  VectorParamsAs1DForOutWhenUnconnected=off
  wires:
  Bus Creator3/1 -> Separator/1
  Purge Rate/1("XMEAS(10) ") -> Bus Creator3/1
  Separator Temperature/1("XMEAS(11) ") -> Bus Creator3/2
  Separator Level/1("XMEAS(12) ") -> Bus Creator3/3
  Separator Pressure/1("XMEAS(13) ") -> Bus Creator3/4
  Separator Underflow/1("XMEAS(14) ") -> Bus Creator3/5

== system COSTEP_Exergy/Process Measurements/Subsystem5 ==
  Bus Creator4 : BusCreator  Inputs=5
  Stripper Level : Subsystem
  Stripper Pressure : Subsystem
  Stripper Steam Flow : Subsystem
  Stripper Temperature : Subsystem
  Stripper Underflow : Subsystem
  Stripper : Outport  VectorParamsAs1DForOutWhenUnconnected=off
  wires:
  Stripper Level/1("XMEAS(15) ") -> Bus Creator4/1
  Bus Creator4/1 -> Stripper/1
  Stripper Steam Flow/1("XMEAS(19) ") -> Bus Creator4/5
  Stripper Temperature/1("XMEAS(18) ") -> Bus Creator4/4
  Stripper Pressure/1("XMEAS(16) ") -> Bus Creator4/2
  Stripper Underflow/1("XMEAS(17) ") -> Bus Creator4/3

== system COSTEP_Exergy/Random number generator/Disturbances 17, 18, 20 IDVWLK=10-12 ==
  G1 : Inport
  Bus Creator : BusCreator  Inputs=3
  Bus Selector : BusSelector  OutputSignals=IDV(17),IDV(18),IDV(20)
  IDVWLK(10) : Gain
  IDVWLK(11) : Gain
  IDVWLK(12) : Gain
  Subsystem1 : Subsystem
  Subsystem10 : Subsystem
  Subsystem2 : Subsystem
  G2 : Outport  VectorParamsAs1DForOutWhenUnconnected=off
  Out1 : Outport  Port=2
  wires:
  Subsystem2/2(G_NEW) -> G2/1
  Subsystem10/2(G_NEW) -> Subsystem1/2(G)
  Bus Creator/1 -> Out1/1
  G1/1 -> Subsystem10/2(G)
  Subsystem10/1(TESUB8(10,Time)) -> Bus Creator/1  "TESUB8(10)"
  Subsystem1/2(G_NEW) -> Subsystem2/2(G)
  [IDV] -> Bus Selector/1
  Bus Selector/1 -> IDVWLK(10)/1  "<IDV(17)>"
  Bus Selector/2 -> IDVWLK(11)/1  "<IDV(18)>"
  Bus Selector/3 -> IDVWLK(12)/1  "<IDV(20)>"
  IDVWLK(10)/1 -> Subsystem10/1(IDVWLK(10))  "IDVWLK(10)"
  IDVWLK(11)/1 -> Subsystem1/1(IDVWLK(11))  "IDVWLK(11)"
  IDVWLK(12)/1 -> Subsystem2/1(IDVWLK(12))  "IDVWLK(12)"
  Subsystem1/1(TESUB8(11,Time)) -> Bus Creator/2  "TESUB8(11)"
  Subsystem2/1(TESUB8(12,Time)) -> Bus Creator/3  "TESUB8(12)"

== system COSTEP_Exergy/Random number generator/Disturbances 21, 22, 23, 24, 25, 26, 27, 28 IDVWLK=13-20 ==
  G : Inport
  Bus Creator : BusCreator  Inputs=8
  Bus Selector1 : BusSelector  OutputSignals=IDV(21),IDV(22),IDV(23),IDV(24),IDV(25),IDV(26),IDV(27),IDV(28)
  IDVWLK(13) : Gain
  IDVWLK(14) : Gain
  IDVWLK(15) : Gain
  IDVWLK(16) : Gain
  IDVWLK(17) : Gain
  IDVWLK(18) : Gain
  IDVWLK(19) : Gain
  IDVWLK(20) : Gain
  Subsystem1 : Subsystem
  Subsystem10 : Subsystem
  Subsystem2 : Subsystem
  Subsystem3 : Subsystem
  Subsystem4 : Subsystem
  Subsystem5 : Subsystem
  Subsystem6 : Subsystem
  Subsystem7 : Subsystem
  G1 : Outport  VectorParamsAs1DForOutWhenUnconnected=off
  Out1 : Outport  Port=2
  wires:
  IDVWLK(13)/1 -> Subsystem10/1(IDVWLK(13))  "IDVWLK(13)"
  G/1 -> Subsystem10/2(G)
  Subsystem6/1(TESUB8(19,Time)) -> Bus Creator/7  "TESUB8(19)"
  Subsystem1/2(G_NEW) -> Subsystem2/2(G)
  Bus Selector1/1 -> IDVWLK(13)/1  "<IDV(21)>"
  Subsystem7/2(G_NEW) -> G1/1
  Subsystem4/1(TESUB8(17,Time)) -> Bus Creator/5  "TESUB8(17)"
  Subsystem5/1(TESUB8(18,Time)) -> Bus Creator/6  "TESUB8(18)"
  Bus Selector1/5 -> IDVWLK(17)/1  "<IDV(25)>"
  IDVWLK(17)/1 -> Subsystem4/1(IDVWLK(17))  "IDVWLK(17)"
  Bus Selector1/7 -> IDVWLK(19)/1  "<IDV(27)>"
  Bus Selector1/4 -> IDVWLK(16)/1  "<IDV(24)>"
  Subsystem5/2(G_NEW) -> Subsystem6/2(G)
  Subsystem3/2(G_NEW) -> Subsystem4/2(G)
  Subsystem7/1(TESUB8(8,Time)) -> Bus Creator/8  "TESUB8(20)"
  Bus Selector1/2 -> IDVWLK(14)/1  "<IDV(22)>"
  Bus Selector1/6 -> IDVWLK(18)/1  "<IDV(26)>"
  [IDV] -> Bus Selector1/1
  Subsystem4/2(G_NEW) -> Subsystem5/2(G)
  IDVWLK(18)/1 -> Subsystem5/1(IDVWLK(18))  "IDVWLK(18)"
  IDVWLK(14)/1 -> Subsystem1/1(IDVWLK(14))  "IDVWLK(14)"
  Subsystem10/1(TESUB8(13,Time)) -> Bus Creator/1  "TESUB8(13)"
  Bus Selector1/3 -> IDVWLK(15)/1  "<IDV(23)>"
  Subsystem2/2(G_NEW) -> Subsystem3/2(G)
  IDVWLK(15)/1 -> Subsystem2/1(IDVWLK(15))  "IDVWLK(15)"
  Subsystem3/1(TESUB8(16,Time)) -> Bus Creator/4  "TESUB8(16)"
  Subsystem6/2(G_NEW) -> Subsystem7/2(G)
  Subsystem2/1(TESUB8(15,Time)) -> Bus Creator/3  "TESUB8(15)"
  Subsystem1/1(TESUB8(14,Time)) -> Bus Creator/2  "TESUB8(14)"
  IDVWLK(20)/1 -> Subsystem7/1(IDVWLK(20))  "IDVWLK(20)"
  Bus Creator/1 -> Out1/1
  Subsystem10/2(G_NEW) -> Subsystem1/2(G)
  Bus Selector1/8 -> IDVWLK(20)/1  "<IDV(28)>"
  IDVWLK(19)/1 -> Subsystem6/1(IDVWLK(19))  "IDVWLK(19)"
  IDVWLK(16)/1 -> Subsystem3/1(IDVWLK(16))  "IDVWLK(16)"

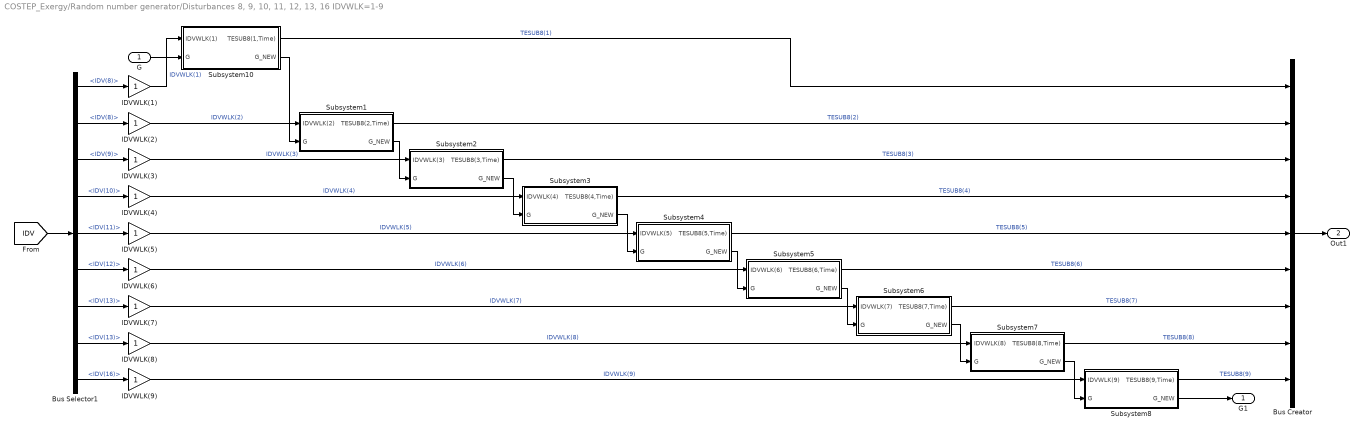
== system COSTEP_Exergy/Random number generator/Disturbances 8, 9, 10, 11, 12, 13, 16 IDVWLK=1-9 ==
  G : Inport
  Bus Creator : BusCreator  Inputs=9
  Bus Selector1 : BusSelector  OutputSignals=IDV(8),IDV(8),IDV(9),IDV(10),IDV(11),IDV(12),IDV(13),IDV(13),IDV(16)
  IDVWLK(1) : Gain
  IDVWLK(2) : Gain
  IDVWLK(3) : Gain
  IDVWLK(4) : Gain
  IDVWLK(5) : Gain
  IDVWLK(6) : Gain
  IDVWLK(7) : Gain
  IDVWLK(8) : Gain
  IDVWLK(9) : Gain
  Subsystem1 : Subsystem
  Subsystem10 : Subsystem
  Subsystem2 : Subsystem
  Subsystem3 : Subsystem
  Subsystem4 : Subsystem
  Subsystem5 : Subsystem
  Subsystem6 : Subsystem
  Subsystem7 : Subsystem
  Subsystem8 : Subsystem
  G1 : Outport  VectorParamsAs1DForOutWhenUnconnected=off
  Out1 : Outport  Port=2
  wires:
  G/1 -> Subsystem10/2(G)
  [IDV] -> Bus Selector1/1
  IDVWLK(4)/1 -> Subsystem3/1(IDVWLK(4))  "IDVWLK(4)"
  Bus Selector1/8 -> IDVWLK(8)/1  "<IDV(13)>"
  IDVWLK(8)/1 -> Subsystem7/1(IDVWLK(8))  "IDVWLK(8)"
  IDVWLK(5)/1 -> Subsystem4/1(IDVWLK(5))  "IDVWLK(5)"
  IDVWLK(3)/1 -> Subsystem2/1(IDVWLK(3))  "IDVWLK(3)"
  Bus Selector1/3 -> IDVWLK(3)/1  "<IDV(9)>"
  IDVWLK(2)/1 -> Subsystem1/1(IDVWLK(2))  "IDVWLK(2)"
  Bus Selector1/6 -> IDVWLK(6)/1  "<IDV(12)>"
  Bus Selector1/4 -> IDVWLK(4)/1  "<IDV(10)>"
  IDVWLK(9)/1 -> Subsystem8/1(IDVWLK(9))  "IDVWLK(9)"
  IDVWLK(6)/1 -> Subsystem5/1(IDVWLK(6))  "IDVWLK(6)"
  IDVWLK(7)/1 -> Subsystem6/1(IDVWLK(7))  "IDVWLK(7)"
  Bus Selector1/9 -> IDVWLK(9)/1  "<IDV(16)>"
  Bus Selector1/5 -> IDVWLK(5)/1  "<IDV(11)>"
  Bus Selector1/7 -> IDVWLK(7)/1  "<IDV(13)>"
  Bus Selector1/2 -> IDVWLK(2)/1  "<IDV(8)>"
  Bus Selector1/1 -> IDVWLK(1)/1  "<IDV(8)>"
  IDVWLK(1)/1 -> Subsystem10/1(IDVWLK(1))  "IDVWLK(1)"
  Subsystem10/2(G_NEW) -> Subsystem1/2(G)
  Subsystem1/2(G_NEW) -> Subsystem2/2(G)
  Subsystem2/2(G_NEW) -> Subsystem3/2(G)
  Subsystem3/2(G_NEW) -> Subsystem4/2(G)
  Subsystem4/2(G_NEW) -> Subsystem5/2(G)
  Subsystem5/2(G_NEW) -> Subsystem6/2(G)
  Subsystem6/2(G_NEW) -> Subsystem7/2(G)
  Subsystem7/2(G_NEW) -> Subsystem8/2(G)
  Subsystem8/2(G_NEW) -> G1/1
  Bus Creator/1 -> Out1/1
  Subsystem10/1(TESUB8(1,Time)) -> Bus Creator/1  "TESUB8(1)"
  Subsystem1/1(TESUB8(2,Time)) -> Bus Creator/2  "TESUB8(2)"
  Subsystem2/1(TESUB8(3,Time)) -> Bus Creator/3  "TESUB8(3)"
  Subsystem3/1(TESUB8(4,Time)) -> Bus Creator/4  "TESUB8(4)"
  Subsystem4/1(TESUB8(5,Time)) -> Bus Creator/5  "TESUB8(5)"
  Subsystem5/1(TESUB8(6,Time)) -> Bus Creator/6  "TESUB8(6)"
  Subsystem6/1(TESUB8(7,Time)) -> Bus Creator/7  "TESUB8(7)"
  Subsystem7/1(TESUB8(8,Time)) -> Bus Creator/8  "TESUB8(8)"
  Subsystem8/1(TESUB8(9,Time)) -> Bus Creator/9  "TESUB8(9)"

== system COSTEP_Exergy/Random number generator/Process Measurements XMEAS(I) I=1-22 ==
  G2 : Inport
  Clock3 : Clock
  Constant : Constant  Value=XNS
  Delay : Delay  DelayLength=1  InitialCondition=0
  MATLAB Function : MATLAB Function  TreatAsAtomicUnit=on
  Subsystem : Subsystem
  G3 : Outport  VectorParamsAs1DForOutWhenUnconnected=off
  tag scope: XMNS=global
  wires:
  Clock3/1 -> MATLAB Function/4(Time)
  [ISD] -> MATLAB Function/3(ISD)
  MATLAB Function/1(G) -> G3/1
  G2/1 -> MATLAB Function/2("G ")
  Constant/1 -> MATLAB Function/1(XNS)
  Subsystem/1("XMNS ") -> [XMNS]
  Delay/1 -> Subsystem/1(XMNS)
  MATLAB Function/2(XMNS) -> Delay/1

== system COSTEP_Exergy/Random number generator/Process Measurements XMEAS(I) I=23-36 ==
  G3 : Inport  SampleTime=0.1
  Clock : Clock
  Constant : Constant  Value=XNS2  SampleTime=0.1
  Delay : Delay  DelayLength=1  InitialCondition=zeros(14,1)
  MATLAB Function : MATLAB Function  TreatAsAtomicUnit=on
  Subsystem : Subsystem
  G4 : Outport  VectorParamsAs1DForOutWhenUnconnected=off
  tag scope: XMNS2=global
  wires:
  MATLAB Function/1(G) -> G4/1
  Subsystem/1("XMNS ") -> [XMNS2]
  G3/1 -> MATLAB Function/2("G ")
  MATLAB Function/2(XMNS) -> Delay/1, Subsystem/1(XMNS)
  Constant/1 -> MATLAB Function/1(XNS)
  Clock/1 -> MATLAB Function/3(TIME)
  Delay/1 -> MATLAB Function/4("XMNS ")

== system COSTEP_Exergy/Random number generator/Process Measurements XMEAS(I) I=37-41 ==
  G4 : Inport
  Clock : Clock
  Constant : Constant  Value=XNS3
  Delay : Delay  DelayLength=1  InitialCondition=zeros(5,1)
  MATLAB Function : MATLAB Function  TreatAsAtomicUnit=on
  Subsystem : Subsystem
  G5 : Outport
  tag scope: XMNS3=global
  wires:
  Subsystem/1("XMNS ") -> [XMNS3]
  MATLAB Function/2(XMNS) -> Delay/1, Subsystem/1(XMNS)
  Constant/1 -> MATLAB Function/1(XNS)
  G4/1 -> MATLAB Function/2("G ")
  MATLAB Function/1(G) -> G5/1
  Clock/1 -> MATLAB Function/3(TIME)
  Delay/1 -> MATLAB Function/4("XMNS ")

== system COSTEP_Exergy/Random number generator/Stream Measurements SMEAS Gas analysis1 ==
  GE2 : Inport
  Gas Analysis Delay : Subsystem
  If Action Subsystem3 : Subsystem  TreatAsAtomicUnit=on
  Subsystem : Subsystem
  GE3 : Outport  VectorParamsAs1DForOutWhenUnconnected=off
  tag scope: XMNSE2=global
  wires:
  GE2/1 -> Subsystem/2(GE2), If Action Subsystem3/1(GE2)
  Subsystem/1(GE3) -> GE3/1
  If Action Subsystem3/2(GE3) -> Subsystem/1(In2)
  Gas Analysis Delay/1(IF(TGAS)) -> If Action Subsystem3/Action
  If Action Subsystem3/1(XMNS) -> [XMNSE2]
